simulink model "RG_Kessler_MCC"  (R2023b)
settings: Solver=VariableStepAuto  StartTime=0.0  StopTime=10.0  RelTol=1e-3
values from neighbouring files (symbols this model uses):
  J = (km*ke*Tm)/Ra    (= 0.0225770865363)    [ProiectSACAPCuCalcule.m]
  ke = en/omegaan    (= 0.383940790552)    [ProiectSACAPCuCalcule.m]
  kE = uan/ucn    (= 28.5714285714)    [ProiectSACAPCuCalcule.m]
  kf = (alfa*mn)/omegaan    (= 0.000916591120063)    [ProiectSACAPCuCalcule.m]
  km = mn/ian    (= 0.383940790552)    [ProiectSACAPCuCalcule.m]
  kMI = 3.5/ian    (= 0.7)    [ProiectSACAPCuCalcule.m]
  kMomega = 5/omegaan    (= 0.0238732414638)    [ProiectSACAPCuCalcule.m]
  kr = 1/(2*kPC*Tsuma)    (= 3.51804123711)    [ProiectSACAPCuCalcule.m]
  ms = mn-mf    (= 1.72773355748)    [ProiectSACAPCuCalcule.m]
  Ra = deltau/ian    (= 3.9175257732)    [ProiectSACAPCuCalcule.m]
  Ta = 0.08    [ProiectSACAPCuCalcule.m]
  Tniu = 0    [ProiectSACAPCuCalcule.m]
  tr = 8.4*Tsuma    (= 0.672)    [ProiectSACAPCuCalcule.m]
  ucn = 3.5    [ProiectSACAPCuCalcule.m]
settings Model: Creator=bartic  LastModifiedBy=bartic

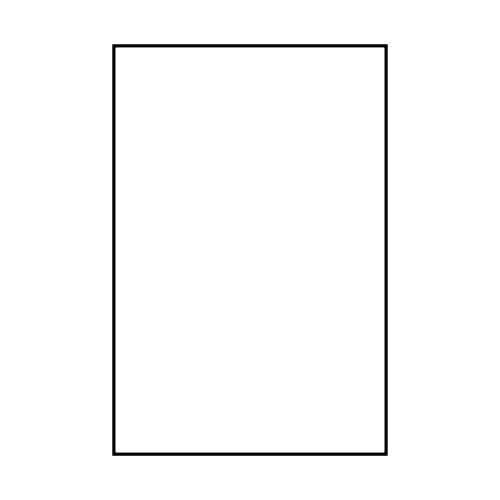
[thumbnail: Simulink's stored preview of the top-level diagram]
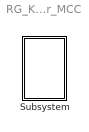
== system RG_Kessler_MCC ==
  Subsystem : Subsystem

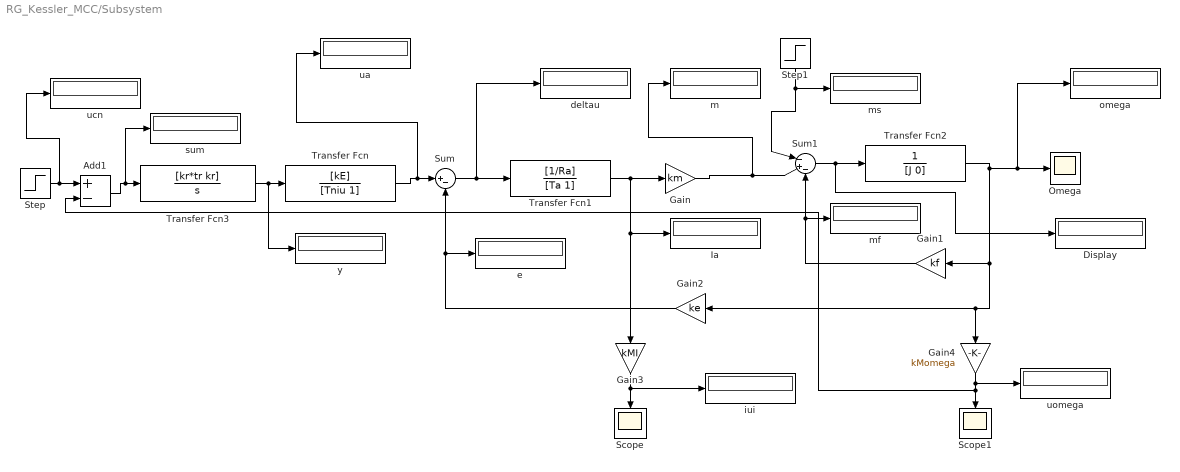
== system RG_Kessler_MCC/Subsystem ==
  Add1 : Sum  Inputs=+-
  Display : Display
  Gain : Gain  Gain=km
  Gain1 : Gain  Gain=kf
  Gain2 : Gain  Gain=ke
  Gain3 : Gain  Gain=kMI
  Gain4 : Gain  Gain=kMomega
  Ia : Display
  Omega : Scope
  Scope : Scope
  Scope1 : Scope
  Step : Step  Time=0  After=ucn  SampleTime=0
  Step1 : Step  Time=0  After=ms  SampleTime=0
  Sum : Sum  Inputs=|+-
  Sum1 : Sum  Inputs=|-+-
  Transfer Fcn : TransferFcn  Numerator=[kE]  Denominator=[Tniu 1]
  Transfer Fcn1 : TransferFcn  Numerator=[1/Ra]  Denominator=[Ta 1]
  Transfer Fcn2 : TransferFcn  Denominator=[J 0]
  Transfer Fcn3 : TransferFcn  Numerator=[kr*tr kr]  Denominator=[1 0]
  deltau : Display
  e : Display
  iui : Display
  m : Display
  mf : Display
  ms : Display
  omega : Display
  sum : Display
  ua : Display
  ucn : Display
  uomega : Display
  y : Display
  wires:
  Transfer Fcn2/1 -> omega/1, Omega/1, Gain4/1, Gain2/1, Gain1/1
  Sum/1 -> deltau/1, Transfer Fcn1/1
  Transfer Fcn1/1 -> Ia/1, Gain3/1, Gain/1
  Step1/1 -> Sum1/1, ms/1
  Transfer Fcn/1 -> ua/1, Sum/1
  Gain/1 -> m/1, Sum1/2
  Gain3/1 -> iui/1, Scope/1
  Gain1/1 -> mf/1, Sum1/3
  Sum1/1 -> Display/1, Transfer Fcn2/1
  Gain2/1 -> e/1, Sum/2
  Gain4/1 -> uomega/1, Add1/2, Scope1/1
  Step/1 -> ucn/1, Add1/1
  Add1/1 -> sum/1, Transfer Fcn3/1
  Transfer Fcn3/1 -> y/1, Transfer Fcn/1
